simulink model "HiPER_SE17"  (R2020b)
settings: Solver=FixedStepAuto  StartTime=0.0  StopTime=20  FixedStep=0.02  RelTol=1e-3
libraries: Lib_EMTAT x21, pid_lib x2
settings Model: Creator=sbianco1  LastModifiedBy=sbianco1

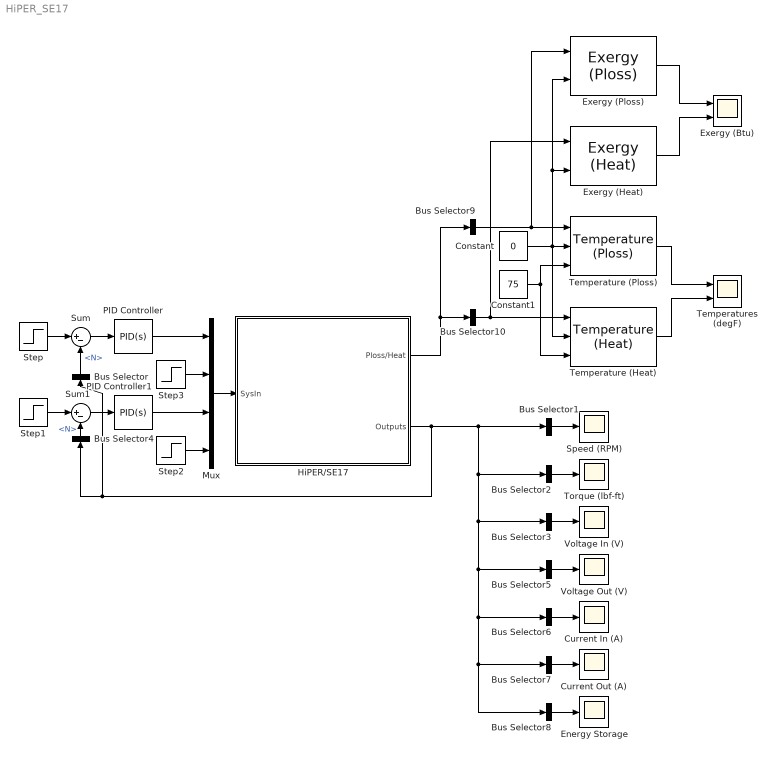
== system HiPER_SE17 ==
  Bus Selector : BusSelector  OutputSignals=S_LS.N
  Bus Selector1 : BusSelector  OutputSignals=S_LS.N,S_HS.N  OutputAsBus=on
  Bus Selector10 : BusSelector  OutputSignals=S_LS,S_HS  OutputAsBus=on
  Bus Selector2 : BusSelector  OutputSignals=M1.T,M2.T,M3.T,M4.T,S_LS.Tnet,S_HS.Tnet  OutputAsBus=on
  Bus Selector3 : BusSelector  OutputSignals=M1.Vin,I1.Vin,C1.Vin,M2.Vin,I2.Vin,C2.Vin,M3.Vin,I3.Vin,C3.Vin,M4.Vin,I4.Vin,C4.Vin,DCDC.Vin,Cap.Vout  OutputAsBus=on
  Bus Selector4 : BusSelector  OutputSignals=S_HS.N
  Bus Selector5 : BusSelector  OutputSignals=I1.Vout,C1.Vout,I2.Vout,C2.Vout,I3.Vout,C3.Vout,I4.Vout,C4.Vout,DCDC.Vout,Cap.Vout  OutputAsBus=on
  Bus Selector6 : BusSelector  OutputSignals=M1.Iin,I1.Iin,C1.Iin,M2.Iin,I2.Iin,C2.Iin,M3.Iin,I3.Iin,C3.Iin,M4.Iin,I4.Iin,C4.Iin,DCDC.Iin  OutputAsBus=on
  Bus Selector7 : BusSelector  OutputSignals=I1.Iout,C1.Iout,I2.Iout,C2.Iout,I3.Iout,C3.Iout,I4.Iout,C4.Iout,DCDC.Iout,Cap.Iout  OutputAsBus=on
  Bus Selector8 : BusSelector  OutputSignals=Cap.Energy,Cap.Vout,Cap.SOC  OutputAsBus=on
  Bus Selector9 : BusSelector  OutputSignals=M1,I1,C1,M2,I2,C2,M3,I3,C3,M4,I4,C4,DCDC,Cap  OutputAsBus=on
  Constant : Constant  Value=0
  Constant1 : Constant  Value=75
  Current In (A) : Scope
  Current Out (A) : Scope
  Energy Storage : Scope
  Exergy (Btu) : Scope  NumInputPorts=2
  Exergy (Heat) : Lib_EMTAT/Extras/Exergy (Heat)  m=0  Cp=0
      settings: AttributesFormatString=|
      | Exergy
      | Version: %<LibraryVersion>
  Exergy (Ploss) : Lib_EMTAT/Extras/Exergy (Ploss)  m=0  Cp=0  Qo=0
      settings: AttributesFormatString=|
      | Exergy
      | Version: %<LibraryVersion>
  HiPER/SE17 : Subsystem
  Mux : Mux
  PID Controller : pid_lib/PID Controller  Controller=PID  Form=Parallel  TimeDomain=Continuous-time  UseExternalTs=off  SampleTime=-1  IntegratorMethod=Forward Euler  FilterMethod=Forward Euler  ControllerParametersSource=internal  P=0.05  I=0.01  D=0  UseFilter=on  N=100  TunerSelectOption=Transfer Function Based (PID Tuner App)  InitialConditionSource=internal  InitialConditionForIntegrator=0  InitialConditionForFilter=0  DifferentiatorICPrevScaledInput=0  ExternalReset=none  TrackingMode=off  Kt=1  LimitOutput=off  SatLimitsSource=internal  UpperSaturationLimit=inf  LowerSaturationLimit=-inf  LinearizeAsGain=on  AntiWindupMode=none  Kb=1  POutMin=[]  POutMax=[]  IOutMin=[]  IOutMax=[]  DOutMin=[]  DOutMax=[]  NOutMin=[]  NOutMax=[]  SumOutMin=[]  SumOutMax=[]  SaturationOutMin=[]  SaturationOutMax=[]  PParamMin=[]  PParamMax=[]  IParamMin=[]  IParamMax=[]  DParamMin=[]  DParamMax=[]  NParamMin=[]  NParamMax=[]  KbParamMin=[]  KbParamMax=[]  KtParamMin=[]  KtParamMax=[]  KbOutMin=[]  KbOutMax=[]  KtOutMin=[]  KtOutMax=[]  IntegratorOutMin=[]  IntegratorOutMax=[]  FilterOutMin=[]  FilterOutMax=[]  SumI1OutMin=[]  SumI1OutMax=[]  SumI2OutMin=[]  SumI2OutMax=[]  SumI3OutMin=[]  SumI3OutMax=[]  SumI4OutMin=[]  SumI4OutMax=[]  SumDOutMin=[]  SumDOutMax=[]  DifferentiatorOutMin=[]  DifferentiatorOutMax=[]  FilterDiffOutCoefMin=[]  FilterDiffOutCoefMax=[]  ReciprocalOutMin=[]  ReciprocalOutMax=[]  SumDenOutMin=[]  SumDenOutMax=[]  SumNumOutMin=[]  SumNumOutMax=[]  DivideOutMin=[]  DivideOutMax=[]  UdiffTsProdOutMin=[]  UdiffTsProdOutMax=[]  NTsProdOutMin=[]  NTsProdOutMax=[]  UintegralTsProdOutMin=[]  UintegralTsProdOutMax=[]  UngainTsProdOutMin=[]  UngainTsProdOutMax=[]  IntegratorContinuousStateAttributes=''  IntegratorStateMustResolveToSignalObject=off  IntegratorRTWStateStorageClass=Auto  FilterContinuousStateAttributes=''  FilterStateMustResolveToSignalObject=off  FilterRTWStateStorageClass=Auto  ParallelPVariant=InternalParameters  IdealPVariant=Disabled  IVariant=InternalParameters  DVariant=InternalParameters  IntegratorVariant=Continuous  SatVariant=Disabled  AWVariant=Passthrough  PCopyVariant=Disabled  TRVariant=Disabled  FdbkBlocksVariant=Forward  IdealPFdbkVariant=Disabled  SatFdbkVariant=Disabled  DerivativeFilterVariant=ContFilter  NVariant=InternalParameters  NCopyVariant=Disabled  FilterICVariant=InternalICsFilter  IntegratorICVariant=InternalICs  ExternalResetVariant=Disabled  TRSumVariant=Passthrough  SumFdbkVariant=Disabled  SumVariant=Sum_PID  TsampFilterVariant=InternalTs  TsampNgainVariant=Passthrough  TsampIntegralVariant=Passthrough  ExternalSaturationOutDataTypeStr=Inherit: Same as second input
  PID Controller1 : pid_lib/PID Controller  Controller=PID  Form=Parallel  TimeDomain=Continuous-time  UseExternalTs=off  SampleTime=-1  IntegratorMethod=Forward Euler  FilterMethod=Forward Euler  ControllerParametersSource=internal  P=0.05  I=0.01  D=0  UseFilter=on  N=100  TunerSelectOption=Transfer Function Based (PID Tuner App)  InitialConditionSource=internal  InitialConditionForIntegrator=0  InitialConditionForFilter=0  DifferentiatorICPrevScaledInput=0  ExternalReset=none  TrackingMode=off  Kt=1  LimitOutput=off  SatLimitsSource=internal  UpperSaturationLimit=inf  LowerSaturationLimit=-inf  LinearizeAsGain=on  AntiWindupMode=none  Kb=1  POutMin=[]  POutMax=[]  IOutMin=[]  IOutMax=[]  DOutMin=[]  DOutMax=[]  NOutMin=[]  NOutMax=[]  SumOutMin=[]  SumOutMax=[]  SaturationOutMin=[]  SaturationOutMax=[]  PParamMin=[]  PParamMax=[]  IParamMin=[]  IParamMax=[]  DParamMin=[]  DParamMax=[]  NParamMin=[]  NParamMax=[]  KbParamMin=[]  KbParamMax=[]  KtParamMin=[]  KtParamMax=[]  KbOutMin=[]  KbOutMax=[]  KtOutMin=[]  KtOutMax=[]  IntegratorOutMin=[]  IntegratorOutMax=[]  FilterOutMin=[]  FilterOutMax=[]  SumI1OutMin=[]  SumI1OutMax=[]  SumI2OutMin=[]  SumI2OutMax=[]  SumI3OutMin=[]  SumI3OutMax=[]  SumI4OutMin=[]  SumI4OutMax=[]  SumDOutMin=[]  SumDOutMax=[]  DifferentiatorOutMin=[]  DifferentiatorOutMax=[]  FilterDiffOutCoefMin=[]  FilterDiffOutCoefMax=[]  ReciprocalOutMin=[]  ReciprocalOutMax=[]  SumDenOutMin=[]  SumDenOutMax=[]  SumNumOutMin=[]  SumNumOutMax=[]  DivideOutMin=[]  DivideOutMax=[]  UdiffTsProdOutMin=[]  UdiffTsProdOutMax=[]  NTsProdOutMin=[]  NTsProdOutMax=[]  UintegralTsProdOutMin=[]  UintegralTsProdOutMax=[]  UngainTsProdOutMin=[]  UngainTsProdOutMax=[]  IntegratorContinuousStateAttributes=''  IntegratorStateMustResolveToSignalObject=off  IntegratorRTWStateStorageClass=Auto  FilterContinuousStateAttributes=''  FilterStateMustResolveToSignalObject=off  FilterRTWStateStorageClass=Auto  ParallelPVariant=InternalParameters  IdealPVariant=Disabled  IVariant=InternalParameters  DVariant=InternalParameters  IntegratorVariant=Continuous  SatVariant=Disabled  AWVariant=Passthrough  PCopyVariant=Disabled  TRVariant=Disabled  FdbkBlocksVariant=Forward  IdealPFdbkVariant=Disabled  SatFdbkVariant=Disabled  DerivativeFilterVariant=ContFilter  NVariant=InternalParameters  NCopyVariant=Disabled  FilterICVariant=InternalICsFilter  IntegratorICVariant=InternalICs  ExternalResetVariant=Disabled  TRSumVariant=Passthrough  SumFdbkVariant=Disabled  SumVariant=Sum_PID  TsampFilterVariant=InternalTs  TsampNgainVariant=Passthrough  TsampIntegralVariant=Passthrough  ExternalSaturationOutDataTypeStr=Inherit: Same as second input
  Speed (RPM) : Scope
  Step : Step  Time=2  After=4000  SampleTime=0
  Step1 : Step  After=4000  SampleTime=0
  Step2 : Step  Time=10  After=50  SampleTime=0
  Step3 : Step  Time=15  After=-50  SampleTime=0
  Sum : Sum  Inputs=|+-
  Sum1 : Sum  Inputs=|+-
  Temperature (Heat) : Lib_EMTAT/Extras/Temperature (Heat)  m=50*ones(2,1)  Cp=0.220*ones(2,1)
      settings: AttributesFormatString=|
      | Temperature
      | Version: %<LibraryVersion>
  Temperature (Ploss) : Lib_EMTAT/Extras/Temperature (Ploss)  m=50*ones(14,1)  Cp=0.220*ones(14,1)  Qo=0*ones(14,1)
      settings: AttributesFormatString=|
      | Temperature
      | Version: %<LibraryVersion>
  Temperatures (degF) : Scope  NumInputPorts=2
  Torque (lbf-ft) : Scope
  Voltage In (V) : Scope
  Voltage Out (V) : Scope
  wires:
  Mux/1 -> HiPER/SE17/1(SysIn)
  PID Controller/1 -> Mux/1
  Sum/1 -> PID Controller/1
  Step/1 -> Sum/1
  Bus Selector/1 -> Sum/2  "<N>"
  Step3/1 -> Mux/2
  Bus Selector1/1 -> Speed (RPM)/1
  Bus Selector2/1 -> Torque (lbf-ft)/1
  Bus Selector3/1 -> Voltage In (V)/1
  Sum1/1 -> PID Controller1/1
  Step1/1 -> Sum1/1
  PID Controller1/1 -> Mux/3
  Bus Selector4/1 -> Sum1/2  "<N>"
  Step2/1 -> Mux/4
  Bus Selector5/1 -> Voltage Out (V)/1
  Bus Selector7/1 -> Current Out (A)/1
  Bus Selector6/1 -> Current In (A)/1
  HiPER/SE17/2(Outputs) -> Bus Selector4/1, Bus Selector/1, Bus Selector7/1, Bus Selector8/1, Bus Selector6/1, Bus Selector5/1, Bus Selector3/1, Bus Selector2/1, Bus Selector1/1
  Bus Selector8/1 -> Energy Storage/1
  Temperature (Ploss)/1 -> Temperatures (degF)/1
  Temperature (Heat)/1 -> Temperatures (degF)/2
  Bus Selector9/1 -> Exergy (Ploss)/1, Temperature (Ploss)/1
  Constant1/1 -> Temperature (Ploss)/3, Temperature (Heat)/3
  HiPER/SE17/1(Ploss/Heat) -> Bus Selector10/1, Bus Selector9/1
  Bus Selector10/1 -> Exergy (Heat)/1, Temperature (Heat)/1
  Constant/1 -> Exergy (Ploss)/2, Exergy (Heat)/2, Temperature (Heat)/2, Temperature (Ploss)/2
  Exergy (Ploss)/1 -> Exergy (Btu)/1
  Exergy (Heat)/1 -> Exergy (Btu)/2

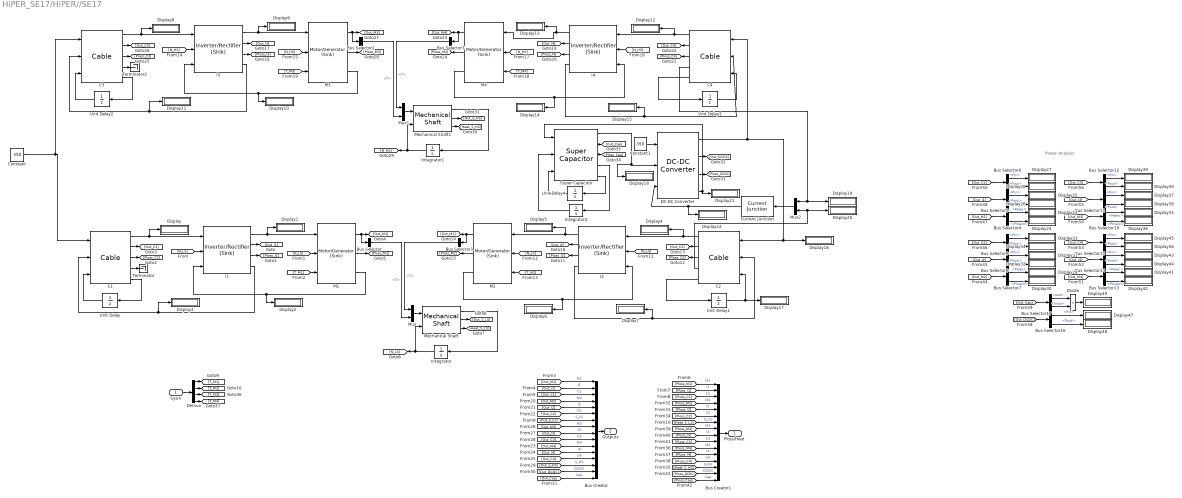
== system HiPER_SE17/HiPER//SE17 ==
  note: Power Analysis
  SysIn : Inport
  Bus Creator : BusCreator  Inputs=16
  Bus Creator1 : BusCreator  Inputs=16
  Bus Selector{,1..3} (4 alike) : BusSelector  OutputSignals=T
  Bus Selector{4,7,10,13} (4 alike) : BusSelector  OutputSignals=Pelec,Pmech
  Bus Selector{5..6,8..9,11..12,14..16} (9 alike) : BusSelector  OutputSignals=Pin,Pout
  Bus Selector17 : BusSelector  OutputSignals=Iout,Vout
  C{1..4} (4 alike) : Lib_EMTAT/Components/Power Flow/Cable  R_c=0.001
      settings: AttributesFormatString=|
      | Cable
      | Version: %<LibraryVersion>
  Constant : Constant  Value=350
  Constant1 : Constant  Value=350
  Current Junction : Lib_EMTAT/Components/Power Flow/Current Junction
      settings: AttributesFormatString=|
      | Current Junction
      | Version: %<LibraryVersion>
  DC-DC Converter : Lib_EMTAT/Components/Power Flow/DC-DC Converter  X_Vin_VoltageVec_M=[0 100 1000 5000]  Y_Iout_CurrentVec_M=[0 10 100 150]  T_C_EffArray_M=0.98*ones(4,4)
      settings: AttributesFormatString=|
      | DC-DC Converter
      | Version: %<LibraryVersion>
  Demux : Demux
  Display{,1..49} (50 alike) : Display
  Divide : Product  Inputs=**
  I{1..4} (4 alike) : Lib_EMTAT/Components/Power Flow/Inverter//Rectifier (Sink)  X_C_VoltageVec_M=[0 100 1000 5000]  Y_C_CurrentVec_M=[0 10 100 150]  T_C_EffArray_M=.90*ones(4,4)  K_e=0.0503
      settings: AttributesFormatString=|
      | Inverter/Rectifier (Sink)
      | Version: %<LibraryVersion>
  Integrator : Integrator
  Integrator1 : Integrator
  Integrator2 : Integrator  InitialCondition=150
  M{1..4} (4 alike) : Lib_EMTAT/Components/Power Flow/Motor//Generator (Sink)  X_C_SpeedVec_M=[0 100 1000 5000]  Y_C_TorqueVec_M=[0 10 100 150]  T_C_EffArray_M=0.99*ones(4,4)
      settings: AttributesFormatString=|
      | Motor/Generator (Sink)
      | Version: %<LibraryVersion>
  Mechanical Shaft : Lib_EMTAT/Components/Power Flow/Mechanical Shaft  J=0.01  B=0.001
      settings: AttributesFormatString=|
      | Mechanical Shaft
      | Version: %<LibraryVersion>
  Mechanical Shaft1 : Lib_EMTAT/Components/Power Flow/Mechanical Shaft  J=0.01  B=0.001
      settings: AttributesFormatString=|
      | Mechanical Shaft
      | Version: %<LibraryVersion>
  Mux : Mux  Inputs=2
  Mux1 : Mux  Inputs=2
  Mux2 : Mux  Inputs=2
  Super Capacitor : Lib_EMTAT/Components/Power Flow/Super Capacitor  C=130  ESR=0.02  ILeak=0  TSE=69
      settings: AttributesFormatString=|
      | Super Capacitor
      | Version: %<LibraryVersion>
  Terminator : Terminator
  Terminator2 : Terminator
  Unit Delay{,1..4} (5 alike) : UnitDelay  SampleTime=-1  HasFrameUpgradeWarning=on
  Ploss/Heat : Outport
  Outputs : Outport  Port=2
  wires:
  I1/3 -> [Ploss_I1]
  [T_M2] -> M2/3
  C4/1 -> Display12/1, I4/1
  I4/1 -> Display13/1, M4/1
  [N_LS] -> M2/2
  C1/4 -> Terminator/1
  C2/5 -> Unit Delay1/1
  M1/3 -> Display2/1, I1/3
  I2/2 -> [Out_I2]
  M1/2 -> [Ploss_M1]
  I1/4 -> Display3/1, C1/2
  Super Capacitor/3 -> [Ploss_Cap]
  I3/2 -> [Out_I3]
  SysIn/1 -> Demux/1
  [N_HS] -> I3/2
  Current Junction/1 -> Display22/1, DC-DC Converter/3
  Demux/2 -> [T_M2]
  I2/4 -> Display7/1, C2/2
  Demux/1 -> [T_M1]
  Constant1/1 -> DC-DC Converter/1
  Unit Delay3/1 -> C4/3
  C1/5 -> Unit Delay/1
  Integrator/1 -> [N_LS], Mechanical Shaft/2
  C1/1 -> Display/1, I1/1
  [N_LS] -> I2/2
  C3/2 -> [Out_C3]
  I2/1 -> Display5/1, M2/1
  Mechanical Shaft1/3 -> [Heat_S_HS]
  C3/3 -> [Ploss_C3]
  Mux1/1 -> Mechanical Shaft1/1
  Super Capacitor/4 -> Integrator2/1
  M4/3 -> I4/3, Display14/1
  [N_LS] -> M1/2
  [T_M3] -> M3/3
  I2/3 -> [Ploss_I2]
  [T_M1] -> M1/3
  Unit Delay2/1 -> C3/3
  M2/1 -> Bus Selector1/1, [Out_M2]
  I1/1 -> Display1/1, M1/1
  I3/3 -> [Ploss_I3]
  Bus Selector3/1 -> Mux1/1  "<T>"
  Unit Delay/1 -> C1/3
  Mechanical Shaft1/2 -> [Out_S_HS]
  Mechanical Shaft/2 -> [Out_S_LS]
  DC-DC Converter/1 -> C2/1, Display16/1, C4/1
  M2/2 -> [Ploss_M2]
  C2/1 -> Display4/1, I2/1
  Integrator1/1 -> [N_HS], Mechanical Shaft1/2
  Bus Selector/1 -> Mux/2  "<T>"
  Mechanical Shaft1/1 -> Integrator1/1
  Constant/1 -> C3/1, C1/1
  Super Capacitor/1 -> Display18/1, DC-DC Converter/2
  DC-DC Converter/4 -> Super Capacitor/1, Display21/1
  Integrator2/1 -> Super Capacitor/2
  M1/1 -> Bus Selector/1, [Out_M1]
  M2/3 -> I2/3, Display6/1
  I4/4 -> Display15/1, C4/2
  Demux/3 -> [T_M3]
  I3/4 -> Display11/1, C3/2
  C2/2 -> [Out_C2]
  C2/3 -> [Ploss_C2]
  DC-DC Converter/2 -> [Out_DCDC]
  DC-DC Converter/3 -> [Ploss_DCDC]
  Unit Delay4/1 -> Super Capacitor/3
  [N_LS] -> I1/2
  Mechanical Shaft/3 -> [Heat_S_LS]
  Mux/1 -> Mechanical Shaft/1
  Unit Delay1/1 -> Display17/1, C2/3
  Mux2/1 -> Current Junction/1
  C2/4 -> Mux2/2, Display20/1
  Demux/4 -> [T_M4]
  Bus Selector1/1 -> Mux/1  "<T>"
  Super Capacitor/5 -> Unit Delay4/1
  I3/1 -> Display9/1, M3/1
  M4/2 -> [Ploss_M4]
  Bus Selector2/1 -> Mux1/2  "<T>"
  M4/1 -> Bus Selector3/1, [Out_M4]
  I4/3 -> [Ploss_I4]
  M3/1 -> Bus Selector2/1, [Out_M3]
  C4/5 -> Unit Delay3/1
  C3/1 -> Display8/1, I3/1
  C3/5 -> Unit Delay2/1
  C3/4 -> Terminator2/1
  M3/3 -> Display10/1, I3/3
  [N_HS] -> M4/2
  I4/2 -> [Out_I4]
  M3/2 -> [Ploss_M3]
  [T_M4] -> M4/3
  C4/3 -> [Ploss_C4]
  C4/2 -> [Out_C4]
  [N_HS] -> I4/2
  [N_HS] -> M3/2
  I1/2 -> [Out_I1]
  Mechanical Shaft/1 -> Integrator/1
  C1/3 -> [Ploss_C1]
  C1/2 -> [Out_C1]
  Super Capacitor/2 -> [Out_Cap]
  [Out_Cap] -> Bus Creator/16  "Cap"
  [Out_DCDC] -> Bus Creator/15  "DCDC"
  [Out_S_HS] -> Bus Creator/14  "S_HS"
  [Out_C4] -> Bus Creator/13  "C4"
  [Out_I4] -> Bus Creator/12  "I4"
  [Out_M4] -> Bus Creator/11  "M4"
  [Out_C3] -> Bus Creator/10  "C3"
  [Out_I3] -> Bus Creator/9  "I3"
  [Out_M3] -> Bus Creator/8  "M3"
  [Out_S_LS] -> Bus Creator/7  "S_LS"
  [Out_C2] -> Bus Creator/6  "C2"
  [Out_I2] -> Bus Creator/5  "I2"
  [Out_M2] -> Bus Creator/4  "M2"
  [Out_C1] -> Bus Creator/3  "C1"
  [Out_I1] -> Bus Creator/2  "I1"
  [Out_M1] -> Bus Creator/1  "M1"
  Bus Creator/1 -> Outputs/1
  Bus Creator1/1 -> Ploss/Heat/1
  [Ploss_C4] -> Bus Creator1/13  "C4"
  [Heat_S_HS] -> Bus Creator1/14  "S_HS"
  [Ploss_DCDC] -> Bus Creator1/15  "DCDC"
  [Ploss_Cap] -> Bus Creator1/16  "Cap"
  [Ploss_I4] -> Bus Creator1/12  "I4"
  [Ploss_M4] -> Bus Creator1/11  "M4"
  [Ploss_C3] -> Bus Creator1/10  "C3"
  [Ploss_I3] -> Bus Creator1/9  "I3"
  [Ploss_M3] -> Bus Creator1/8  "M3"
  [Heat_S_LS] -> Bus Creator1/7  "S_LS"
  [Ploss_C2] -> Bus Creator1/6  "C2"
  [Ploss_I2] -> Bus Creator1/5  "I2"
  [Ploss_M2] -> Bus Creator1/4  "M2"
  [Ploss_C1] -> Bus Creator1/3  "C1"
  [Ploss_I1] -> Bus Creator1/2  "I1"
  [Ploss_M1] -> Bus Creator1/1  "M1"
  C4/4 -> Mux2/1, Display19/1
  [Out_M1] -> Bus Selector4/1
  Bus Selector4/1 -> Display23/1  "<Pelec>"
  Bus Selector4/2 -> Display24/1  "<Pmech>"
  Bus Selector5/2 -> Display26/1  "<Pout>"
  Bus Selector5/1 -> Display25/1  "<Pin>"
  [Out_I1] -> Bus Selector5/1
  [Out_C1] -> Bus Selector6/1
  Bus Selector6/1 -> Display27/1  "<Pin>"
  Bus Selector6/2 -> Display28/1  "<Pout>"
  Bus Selector9/2 -> Display34/1  "<Pout>"
  Bus Selector9/1 -> Display33/1  "<Pin>"
  [Out_C2] -> Bus Selector9/1
  [Out_I2] -> Bus Selector8/1
  Bus Selector8/1 -> Display31/1  "<Pin>"
  Bus Selector8/2 -> Display32/1  "<Pout>"
  Bus Selector7/2 -> Display30/1  "<Pmech>"
  Bus Selector7/1 -> Display29/1  "<Pelec>"
  [Out_M2] -> Bus Selector7/1
  Bus Selector11/2 -> Display38/1  "<Pout>"
  [Out_C3] -> Bus Selector12/1
  [Out_I3] -> Bus Selector11/1
  Bus Selector10/1 -> Display35/1  "<Pelec>"
  Bus Selector10/2 -> Display36/1  "<Pmech>"
  [Out_I4] -> Bus Selector14/1
  Bus Selector13/1 -> Display41/1  "<Pelec>"
  Bus Selector14/1 -> Display43/1  "<Pin>"
  Bus Selector15/1 -> Display45/1  "<Pin>"
  Bus Selector14/2 -> Display44/1  "<Pout>"
  Bus Selector13/2 -> Display42/1  "<Pmech>"
  Bus Selector11/1 -> Display37/1  "<Pin>"
  [Out_M3] -> Bus Selector10/1
  Bus Selector12/2 -> Display40/1  "<Pout>"
  [Out_C4] -> Bus Selector15/1
  Bus Selector12/1 -> Display39/1  "<Pin>"
  Bus Selector15/2 -> Display46/1  "<Pout>"
  [Out_M4] -> Bus Selector13/1
  [Out_Cap] -> Bus Selector17/1
  Bus Selector16/2 -> Display48/1  "<Pout>"
  Bus Selector17/1 -> Divide/1  "<Iout>"
  Bus Selector16/1 -> Display47/1  "<Pin>"
  [Out_DCDC] -> Bus Selector16/1
  Bus Selector17/2 -> Divide/2  "<Vout>"
  Divide/1 -> Display49/1
